simulink model "generate_model_data"  (R2016b)
settings: Solver=VariableStepAuto  StartTime=0.0  StopTime=t(end)  RelTol=1e-3
values from neighbouring files (symbols this model uses):
  A1 = [1.0000   -1.6    0.7]    [examples.m]
  A2 = [1.0000   -1.6    0.7]    [examples.m]
  A3 = [1.0000   -1.6    0.7]    [examples.m]
  A4 = [1.0000   -1.6    0.7]    [examples.m]
  B1 = [0 0 .2]    [examples.m]
  B2 = [0 0 .2]    [examples.m]
  B3 = [0 1 -.2]    [examples.m]
  B4 = [0 1 -.2]    [examples.m]
  C1 = 1    [examples.m]
  C2 = 1    [examples.m]
  C3 = 1    [examples.m]
  C4 = [1 -0.3]    [examples.m]
  D1 = 1    [examples.m]
  D2 = A2    [examples.m]
  D3 = A3    [examples.m]
  D4 = [1 -1]    [examples.m]
  Ts = 0.05    [examples.m]
settings Model: Creator=schauer  LastModifiedBy=schauer

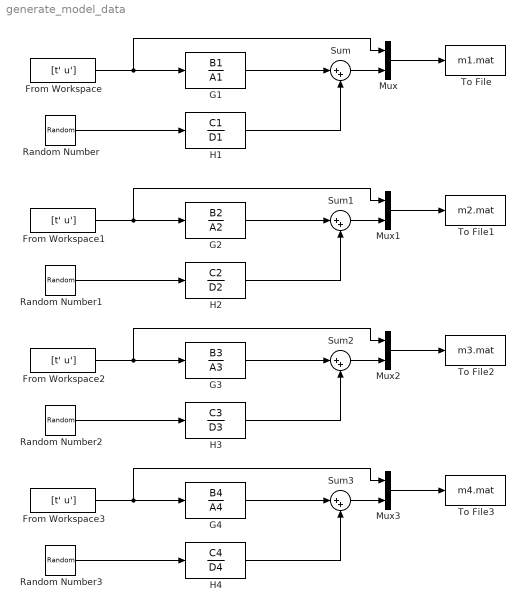
== system generate_model_data ==
  From Workspace{,1..3} (4 alike) : FromWorkspace  VariableName=[t' u']  SampleTime=0  Interpolate=off  OutputAfterFinalValue=Setting to zero
  G1 : DiscreteFilter  Numerator=B1  Denominator=A1  SampleTime=Ts
  G2 : DiscreteFilter  Numerator=B2  Denominator=A2  SampleTime=Ts
  G3 : DiscreteFilter  Numerator=B3  Denominator=A3  SampleTime=Ts
  G4 : DiscreteFilter  Numerator=B4  Denominator=A4  SampleTime=Ts
  H1 : DiscreteFilter  Numerator=C1  Denominator=D1  SampleTime=Ts
  H2 : DiscreteFilter  Numerator=C2  Denominator=D2  SampleTime=Ts
  H3 : DiscreteFilter  Numerator=C3  Denominator=D3  SampleTime=Ts
  H4 : DiscreteFilter  Numerator=C4  Denominator=D4  SampleTime=Ts
  Mux{,1..3} (4 alike) : Mux  Inputs=2
  Random Number{,1..3} (4 alike) : RandomNumber  Variance=0.001  SampleTime=Ts
  Sum{,1..3} (4 alike) : Sum  Inputs=|++
  To File : ToFile  Filename=m1.mat  MatrixName=io_data  SampleTime=Ts
  To File1 : ToFile  Filename=m2.mat  MatrixName=io_data  SampleTime=Ts
  To File2 : ToFile  Filename=m3.mat  MatrixName=io_data  SampleTime=Ts
  To File3 : ToFile  Filename=m4.mat  MatrixName=io_data  SampleTime=Ts
  wires:
  G1/1 -> Sum/1
  H1/1 -> Sum/2
  Mux/1 -> To File/1
  From Workspace/1 -> Mux/1, G1/1
  Sum/1 -> Mux/2
  Random Number/1 -> H1/1
  G2/1 -> Sum1/1
  H2/1 -> Sum1/2
  Mux1/1 -> To File1/1
  From Workspace1/1 -> Mux1/1, G2/1
  Sum1/1 -> Mux1/2
  Random Number1/1 -> H2/1
  G3/1 -> Sum2/1
  H3/1 -> Sum2/2
  Mux2/1 -> To File2/1
  From Workspace2/1 -> Mux2/1, G3/1
  Sum2/1 -> Mux2/2
  Random Number2/1 -> H3/1
  G4/1 -> Sum3/1
  H4/1 -> Sum3/2
  Mux3/1 -> To File3/1
  From Workspace3/1 -> Mux3/1, G4/1
  Sum3/1 -> Mux3/2
  Random Number3/1 -> H4/1
